simulink model "gain_output_controller"  (R2020b)
settings: Solver=FixedStepAuto  StartTime=0.0  StopTime=stop_time  RelTol=1e-3
values from neighbouring files (symbols this model uses):
  accum_delay = max(band_sizes)    [gain_output_controller_sim_init.m]
  accum_delay_memory_size = 2^accum_delay_memory    [gain_output_controller_sim_init.m]
  gainapp_dp_memory = log2(num_bands) + 1    [gain_output_controller_sim_init.m]
libraries: hdlsllib x3
settings Model: Creator=t96f346  LastModifiedBy=conno
settings DataIOCC: SaveOutput=off  SaveTime=off  ReturnWorkspaceOutputs=off
settings OptimizationCC: DefaultParameterBehavior=Inlined
settings ModelReferenceCC: ModelReferenceNumInstancesAllowed=Single

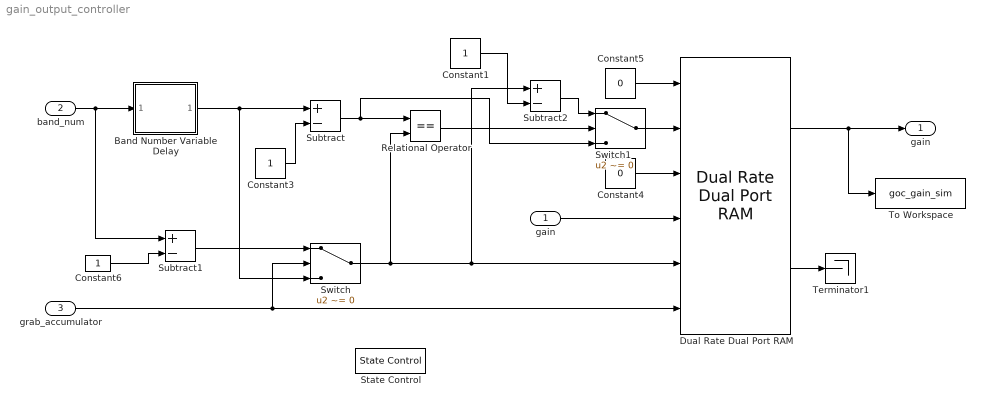
== system gain_output_controller ==
  gain : Inport  OutDataTypeStr=gain_coeff_type  PortDimensions=[1 1]
  band_num : Inport  Port=2  OutDataTypeStr=uint8  PortDimensions=1
  grab_accumulator : Inport  Port=3  OutDataTypeStr=boolean  PortDimensions=1
  Band Number Variable Delay : Subsystem
  Constant1 : Constant  OutDataTypeStr=uint8  SampleTime=-1
  Constant3 : Constant  OutDataTypeStr=uint8  SampleTime=-1
  Constant4 : Constant  Value=0  OutDataTypeStr=boolean  SampleTime=-1
  Constant5 : Constant  Value=0  OutDataTypeStr=fixdt(1,16,8)  SampleTime=-1
  Constant6 : Constant  OutDataTypeStr=Inherit: Inherit via back propagation  SampleTime=-1
  Dual Rate Dual Port RAM : hdlsllib/HDL RAMs/Dual Rate Dual Port RAM  ram_size=gainapp_dp_memory
      settings: SourceProductBaseCode=SL
  Relational Operator : RelationalOperator  Operator===  OutDataTypeStr=boolean  RndMeth=Nearest
  State Control : StateControl  StateControl=Synchronous
  Subtract : Sum  Inputs=+-  OutMin=[0]  OutMax=[2^gainapp_dp_memory-1]  OutDataTypeStr=fixdt(0,gainapp_dp_memory)
  Subtract1 : Sum  Inputs=+-  OutMin=[0]  OutMax=[2^gainapp_dp_memory-1]  OutDataTypeStr=fixdt(0,gainapp_dp_memory)
  Subtract2 : Sum  Inputs=+-  OutMin=[0]  OutMax=[2^gainapp_dp_memory-1]  OutDataTypeStr=fixdt(0,gainapp_dp_memory)
  Switch : Switch  Criteria=u2 ~= 0  OutMin=[0]  OutMax=[2^gainapp_dp_memory-1]  OutDataTypeStr=fixdt(0,gainapp_dp_memory)
  Switch1 : Switch  Criteria=u2 ~= 0
  Terminator1 : Terminator
  To Workspace : ToWorkspace  VariableName=goc_gain_sim  SampleTime=-1
  "gain " : Outport  PortDimensions=1
  wires:
  Subtract2/1 -> Switch1/1
  Relational Operator/1 -> Switch1/2
  Subtract/1 -> Switch1/3, Relational Operator/1
  Constant1/1 -> Subtract2/2
  Switch1/1 -> Dual Rate Dual Port RAM/2
  Switch/1 -> Relational Operator/2, Dual Rate Dual Port RAM/5, Subtract2/1
  band_num/1 -> Band Number Variable Delay/1(data_in), Subtract1/1
  gain/1 -> Dual Rate Dual Port RAM/4
  Dual Rate Dual Port RAM/2 -> Terminator1/1
  Band Number Variable Delay/1(rd_dout) -> Switch/3, Subtract/1
  Subtract1/1 -> Switch/1
  grab_accumulator/1 -> Dual Rate Dual Port RAM/6, Switch/2
  Constant4/1 -> Dual Rate Dual Port RAM/3
  Constant3/1 -> Subtract/2
  Constant6/1 -> Subtract1/2
  Constant5/1 -> Dual Rate Dual Port RAM/1
  Dual Rate Dual Port RAM/1 -> To Workspace/1, "gain "/1

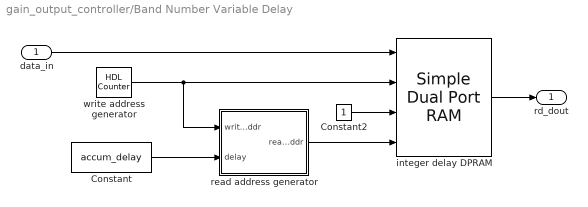
== system gain_output_controller/Band Number Variable Delay ==
  data_in : Inport
  Constant : Constant  Value=accum_delay  OutDataTypeStr=uint8  SampleTime=-1
  Constant2 : Constant  OutDataTypeStr=Inherit: Inherit via back propagation  SampleTime=-1
  integer delay DPRAM : hdlsllib/HDL RAMs/Simple Dual Port RAM  ram_size=accum_delay_memory
      settings: SourceProductBaseCode=SL
  read address generator : Subsystem
  write address generator : hdlsllib/Sources/HDL Counter  CountType=Count limited  CountInit=0  CountStep=1  CountMax=accum_delay_memory_size-1  CountFromType=Initial value  CountFrom=0  CountResetPort=off  CountLoadPort=off  CountEnbPort=off  CountDirPort=off  CountDataType=Unsigned  CountWordLen=accum_delay_memory  CountFracLen=0  CountSampTime=-1
  rd_dout : Outport
  wires:
  Constant2/1 -> integer delay DPRAM/3
  write address generator/1 -> integer delay DPRAM/2, read address generator/1(write_addr)
  integer delay DPRAM/1 -> rd_dout/1
  Constant/1 -> read address generator/2(delay)
  data_in/1 -> integer delay DPRAM/1
  read address generator/1(read_addr) -> integer delay DPRAM/4

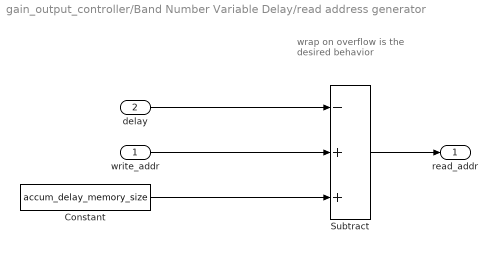
== system gain_output_controller/Band Number Variable Delay/read address generator ==
  note: wrap on overflow is the desired behavior
  write_addr : Inport
  delay : Inport  Port=2
  Constant : Constant  Value=accum_delay_memory_size  OutDataTypeStr=uint8  SampleTime=-1
  Subtract : Sum  Inputs=-++  OutDataTypeStr=Inherit: Inherit via back propagation
  read_addr : Outport  VectorParamsAs1DForOutWhenUnconnected=off
  wires:
  Subtract/1 -> read_addr/1
  write_addr/1 -> Subtract/2
  delay/1 -> Subtract/1
  Constant/1 -> Subtract/3
